simulink library "inp"  (R2024a)
settings: Solver=VariableStepAuto  StartTime=0.0  StopTime=10.0  RelTol=1e-3
undefined symbols (not defined in the file): C_TASK_5MS_S, TRUE
libraries: FVT_lib x54, hcu_lib x1
(part 2 of 2)

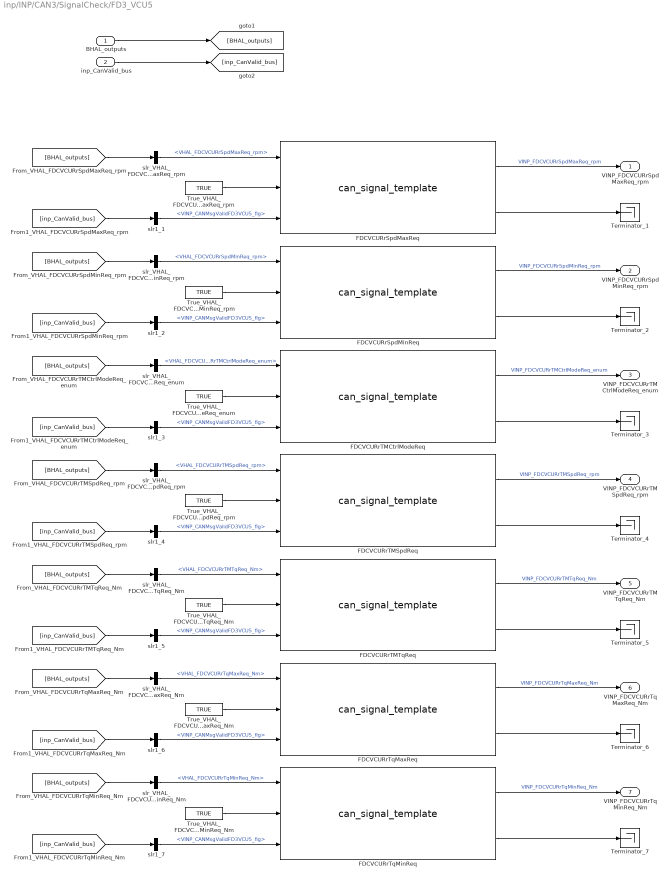
== system inp/INP/CAN3/SignalCheck/FD3_VCU5 ==
  BHAL_outputs : Inport
  inp_CanValid_bus : Inport  Port=2
  FDCVCURrSpdMaxReq : FVT_lib/inp/can_signal_template  SystemSampleTime=-1  VariantActivationTime=update diagram  AllowFlexibleInterface=on  Latency=0  AutoFrameSizeCalculation=off
      link override defval: Value=KINP_FDCVCURrSpdMaxReq_rpm_defval
      link override ovrdflg: Value=KINP_FDCVCURrSpdMaxReq_rpm_ovrdflg
      link override ovrdval: Value=KINP_FDCVCURrSpdMaxReq_rpm_ovrdval
  FDCVCURrSpdMinReq : FVT_lib/inp/can_signal_template  SystemSampleTime=-1  VariantActivationTime=update diagram  AllowFlexibleInterface=on  Latency=0  AutoFrameSizeCalculation=off
      link override defval: Value=KINP_FDCVCURrSpdMinReq_rpm_defval
      link override ovrdflg: Value=KINP_FDCVCURrSpdMinReq_rpm_ovrdflg
      link override ovrdval: Value=KINP_FDCVCURrSpdMinReq_rpm_ovrdval
  FDCVCURrTMCtrlModeReq : FVT_lib/inp/can_signal_template  SystemSampleTime=-1  VariantActivationTime=update diagram  AllowFlexibleInterface=on  Latency=0  AutoFrameSizeCalculation=off
      link override defval: Value=KINP_FDCVCURrTMCtrlModeReq_enum_defval
      link override ovrdflg: Value=KINP_FDCVCURrTMCtrlModeReq_enum_ovrdflg
      link override ovrdval: Value=KINP_FDCVCURrTMCtrlModeReq_enum_ovrdval
  FDCVCURrTMSpdReq : FVT_lib/inp/can_signal_template  SystemSampleTime=-1  VariantActivationTime=update diagram  AllowFlexibleInterface=on  Latency=0  AutoFrameSizeCalculation=off
      link override defval: Value=KINP_FDCVCURrTMSpdReq_rpm_defval
      link override ovrdflg: Value=KINP_FDCVCURrTMSpdReq_rpm_ovrdflg
      link override ovrdval: Value=KINP_FDCVCURrTMSpdReq_rpm_ovrdval
  FDCVCURrTMTqReq : FVT_lib/inp/can_signal_template  SystemSampleTime=-1  VariantActivationTime=update diagram  AllowFlexibleInterface=on  Latency=0  AutoFrameSizeCalculation=off
      link override defval: Value=KINP_FDCVCURrTMTqReq_Nm_defval
      link override ovrdflg: Value=KINP_FDCVCURrTMTqReq_Nm_ovrdflg
      link override ovrdval: Value=KINP_FDCVCURrTMTqReq_Nm_ovrdval
  FDCVCURrTqMaxReq : FVT_lib/inp/can_signal_template  SystemSampleTime=-1  VariantActivationTime=update diagram  AllowFlexibleInterface=on  Latency=0  AutoFrameSizeCalculation=off
      link override defval: Value=KINP_FDCVCURrTqMaxReq_Nm_defval
      link override ovrdflg: Value=KINP_FDCVCURrTqMaxReq_Nm_ovrdflg
      link override ovrdval: Value=KINP_FDCVCURrTqMaxReq_Nm_ovrdval
  FDCVCURrTqMinReq : FVT_lib/inp/can_signal_template  SystemSampleTime=-1  VariantActivationTime=update diagram  AllowFlexibleInterface=on  Latency=0  AutoFrameSizeCalculation=off
      link override defval: Value=KINP_FDCVCURrTqMinReq_Nm_defval
      link override ovrdflg: Value=KINP_FDCVCURrTqMinReq_Nm_ovrdflg
      link override ovrdval: Value=KINP_FDCVCURrTqMinReq_Nm_ovrdval
  Terminator_{1..7} (7 alike) : Terminator
  True_VHAL_FDCVCURrSpdMaxReq_rpm : Constant  Value=TRUE  OutDataTypeStr=boolean
  True_VHAL_FDCVCURrSpdMinReq_rpm : Constant  Value=TRUE  OutDataTypeStr=boolean
  True_VHAL_FDCVCURrTMCtrlModeReq_enum : Constant  Value=TRUE  OutDataTypeStr=boolean
  True_VHAL_FDCVCURrTMSpdReq_rpm : Constant  Value=TRUE  OutDataTypeStr=boolean
  True_VHAL_FDCVCURrTMTqReq_Nm : Constant  Value=TRUE  OutDataTypeStr=boolean
  True_VHAL_FDCVCURrTqMaxReq_Nm : Constant  Value=TRUE  OutDataTypeStr=boolean
  True_VHAL_FDCVCURrTqMinReq_Nm : Constant  Value=TRUE  OutDataTypeStr=boolean
  slr1_{1..7} (7 alike) : BusSelector  OutputSignals=VINP_CANMsgValidFD3VCU5_flg
  slr_VHAL_FDCVCURrSpdMaxReq_rpm : BusSelector  OutputSignals=VHAL_FDCVCURrSpdMaxReq_rpm
  slr_VHAL_FDCVCURrSpdMinReq_rpm : BusSelector  OutputSignals=VHAL_FDCVCURrSpdMinReq_rpm
  slr_VHAL_FDCVCURrTMCtrlModeReq_enum : BusSelector  OutputSignals=VHAL_FDCVCURrTMCtrlModeReq_enum
  slr_VHAL_FDCVCURrTMSpdReq_rpm : BusSelector  OutputSignals=VHAL_FDCVCURrTMSpdReq_rpm
  slr_VHAL_FDCVCURrTMTqReq_Nm : BusSelector  OutputSignals=VHAL_FDCVCURrTMTqReq_Nm
  slr_VHAL_FDCVCURrTqMaxReq_Nm : BusSelector  OutputSignals=VHAL_FDCVCURrTqMaxReq_Nm
  slr_VHAL_FDCVCURrTqMinReq_Nm : BusSelector  OutputSignals=VHAL_FDCVCURrTqMinReq_Nm
  VINP_FDCVCURrSpdMaxReq_rpm : Outport
  VINP_FDCVCURrSpdMinReq_rpm : Outport  Port=2
  VINP_FDCVCURrTMCtrlModeReq_enum : Outport  Port=3
  VINP_FDCVCURrTMSpdReq_rpm : Outport  Port=4
  VINP_FDCVCURrTMTqReq_Nm : Outport  Port=5
  VINP_FDCVCURrTqMaxReq_Nm : Outport  Port=6
  VINP_FDCVCURrTqMinReq_Nm : Outport  Port=7
  wires:
  BHAL_outputs/1 -> [BHAL_outputs]
  inp_CanValid_bus/1 -> [inp_CanValid_bus]
  [BHAL_outputs] -> slr_VHAL_FDCVCURrSpdMaxReq_rpm/1
  slr_VHAL_FDCVCURrSpdMaxReq_rpm/1 -> FDCVCURrSpdMaxReq/1  "<VHAL_FDCVCURrSpdMaxReq_rpm>"
  True_VHAL_FDCVCURrSpdMaxReq_rpm/1 -> FDCVCURrSpdMaxReq/2
  [inp_CanValid_bus] -> slr1_1/1
  slr1_1/1 -> FDCVCURrSpdMaxReq/3  "<VINP_CANMsgValidFD3VCU5_flg>"
  FDCVCURrSpdMaxReq/1 -> VINP_FDCVCURrSpdMaxReq_rpm/1  "VINP_FDCVCURrSpdMaxReq_rpm"
  FDCVCURrSpdMaxReq/2 -> Terminator_1/1
  [BHAL_outputs] -> slr_VHAL_FDCVCURrSpdMinReq_rpm/1
  slr_VHAL_FDCVCURrSpdMinReq_rpm/1 -> FDCVCURrSpdMinReq/1  "<VHAL_FDCVCURrSpdMinReq_rpm>"
  True_VHAL_FDCVCURrSpdMinReq_rpm/1 -> FDCVCURrSpdMinReq/2
  [inp_CanValid_bus] -> slr1_2/1
  slr1_2/1 -> FDCVCURrSpdMinReq/3  "<VINP_CANMsgValidFD3VCU5_flg>"
  FDCVCURrSpdMinReq/1 -> VINP_FDCVCURrSpdMinReq_rpm/1  "VINP_FDCVCURrSpdMinReq_rpm"
  FDCVCURrSpdMinReq/2 -> Terminator_2/1
  [BHAL_outputs] -> slr_VHAL_FDCVCURrTMCtrlModeReq_enum/1
  slr_VHAL_FDCVCURrTMCtrlModeReq_enum/1 -> FDCVCURrTMCtrlModeReq/1  "<VHAL_FDCVCURrTMCtrlModeReq_enum>"
  True_VHAL_FDCVCURrTMCtrlModeReq_enum/1 -> FDCVCURrTMCtrlModeReq/2
  [inp_CanValid_bus] -> slr1_3/1
  slr1_3/1 -> FDCVCURrTMCtrlModeReq/3  "<VINP_CANMsgValidFD3VCU5_flg>"
  FDCVCURrTMCtrlModeReq/1 -> VINP_FDCVCURrTMCtrlModeReq_enum/1  "VINP_FDCVCURrTMCtrlModeReq_enum"
  FDCVCURrTMCtrlModeReq/2 -> Terminator_3/1
  [BHAL_outputs] -> slr_VHAL_FDCVCURrTMSpdReq_rpm/1
  slr_VHAL_FDCVCURrTMSpdReq_rpm/1 -> FDCVCURrTMSpdReq/1  "<VHAL_FDCVCURrTMSpdReq_rpm>"
  True_VHAL_FDCVCURrTMSpdReq_rpm/1 -> FDCVCURrTMSpdReq/2
  [inp_CanValid_bus] -> slr1_4/1
  slr1_4/1 -> FDCVCURrTMSpdReq/3  "<VINP_CANMsgValidFD3VCU5_flg>"
  FDCVCURrTMSpdReq/1 -> VINP_FDCVCURrTMSpdReq_rpm/1  "VINP_FDCVCURrTMSpdReq_rpm"
  FDCVCURrTMSpdReq/2 -> Terminator_4/1
  [BHAL_outputs] -> slr_VHAL_FDCVCURrTMTqReq_Nm/1
  slr_VHAL_FDCVCURrTMTqReq_Nm/1 -> FDCVCURrTMTqReq/1  "<VHAL_FDCVCURrTMTqReq_Nm>"
  True_VHAL_FDCVCURrTMTqReq_Nm/1 -> FDCVCURrTMTqReq/2
  [inp_CanValid_bus] -> slr1_5/1
  slr1_5/1 -> FDCVCURrTMTqReq/3  "<VINP_CANMsgValidFD3VCU5_flg>"
  FDCVCURrTMTqReq/1 -> VINP_FDCVCURrTMTqReq_Nm/1  "VINP_FDCVCURrTMTqReq_Nm"
  FDCVCURrTMTqReq/2 -> Terminator_5/1
  [BHAL_outputs] -> slr_VHAL_FDCVCURrTqMaxReq_Nm/1
  slr_VHAL_FDCVCURrTqMaxReq_Nm/1 -> FDCVCURrTqMaxReq/1  "<VHAL_FDCVCURrTqMaxReq_Nm>"
  True_VHAL_FDCVCURrTqMaxReq_Nm/1 -> FDCVCURrTqMaxReq/2
  [inp_CanValid_bus] -> slr1_6/1
  slr1_6/1 -> FDCVCURrTqMaxReq/3  "<VINP_CANMsgValidFD3VCU5_flg>"
  FDCVCURrTqMaxReq/1 -> VINP_FDCVCURrTqMaxReq_Nm/1  "VINP_FDCVCURrTqMaxReq_Nm"
  FDCVCURrTqMaxReq/2 -> Terminator_6/1
  [BHAL_outputs] -> slr_VHAL_FDCVCURrTqMinReq_Nm/1
  slr_VHAL_FDCVCURrTqMinReq_Nm/1 -> FDCVCURrTqMinReq/1  "<VHAL_FDCVCURrTqMinReq_Nm>"
  True_VHAL_FDCVCURrTqMinReq_Nm/1 -> FDCVCURrTqMinReq/2
  [inp_CanValid_bus] -> slr1_7/1
  slr1_7/1 -> FDCVCURrTqMinReq/3  "<VINP_CANMsgValidFD3VCU5_flg>"
  FDCVCURrTqMinReq/1 -> VINP_FDCVCURrTqMinReq_Nm/1  "VINP_FDCVCURrTqMinReq_Nm"
  FDCVCURrTqMinReq/2 -> Terminator_7/1

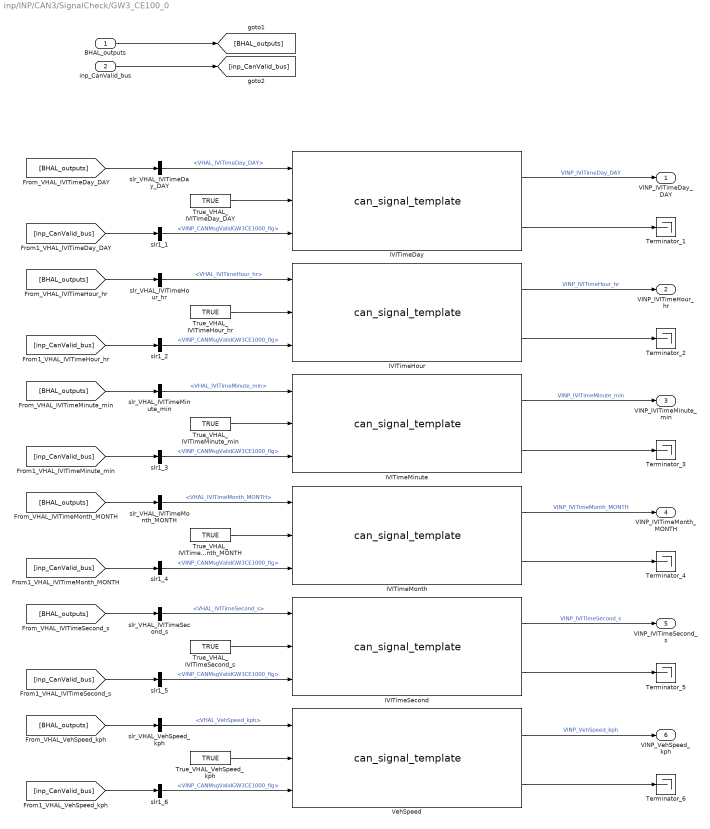
== system inp/INP/CAN3/SignalCheck/GW3_CE100_0 ==
  BHAL_outputs : Inport
  inp_CanValid_bus : Inport  Port=2
  IVITimeDay : FVT_lib/inp/can_signal_template  SystemSampleTime=-1  VariantActivationTime=update diagram  AllowFlexibleInterface=on  Latency=0  AutoFrameSizeCalculation=off
      link override defval: Value=KINP_IVITimeDay_DAY_defval
      link override ovrdflg: Value=KINP_IVITimeDay_DAY_ovrdflg
      link override ovrdval: Value=KINP_IVITimeDay_DAY_ovrdval
  IVITimeHour : FVT_lib/inp/can_signal_template  SystemSampleTime=-1  VariantActivationTime=update diagram  AllowFlexibleInterface=on  Latency=0  AutoFrameSizeCalculation=off
      link override defval: Value=KINP_IVITimeHour_hr_defval
      link override ovrdflg: Value=KINP_IVITimeHour_hr_ovrdflg
      link override ovrdval: Value=KINP_IVITimeHour_hr_ovrdval
  IVITimeMinute : FVT_lib/inp/can_signal_template  SystemSampleTime=-1  VariantActivationTime=update diagram  AllowFlexibleInterface=on  Latency=0  AutoFrameSizeCalculation=off
      link override defval: Value=KINP_IVITimeMinute_min_defval
      link override ovrdflg: Value=KINP_IVITimeMinute_min_ovrdflg
      link override ovrdval: Value=KINP_IVITimeMinute_min_ovrdval
  IVITimeMonth : FVT_lib/inp/can_signal_template  SystemSampleTime=-1  VariantActivationTime=update diagram  AllowFlexibleInterface=on  Latency=0  AutoFrameSizeCalculation=off
      link override defval: Value=KINP_IVITimeMonth_MONTH_defval
      link override ovrdflg: Value=KINP_IVITimeMonth_MONTH_ovrdflg
      link override ovrdval: Value=KINP_IVITimeMonth_MONTH_ovrdval
  IVITimeSecond : FVT_lib/inp/can_signal_template  SystemSampleTime=-1  VariantActivationTime=update diagram  AllowFlexibleInterface=on  Latency=0  AutoFrameSizeCalculation=off
      link override defval: Value=KINP_IVITimeSecond_s_defval
      link override ovrdflg: Value=KINP_IVITimeSecond_s_ovrdflg
      link override ovrdval: Value=KINP_IVITimeSecond_s_ovrdval
  Terminator_{1..6} (6 alike) : Terminator
  True_VHAL_IVITimeDay_DAY : Constant  Value=TRUE  OutDataTypeStr=boolean
  True_VHAL_IVITimeHour_hr : Constant  Value=TRUE  OutDataTypeStr=boolean
  True_VHAL_IVITimeMinute_min : Constant  Value=TRUE  OutDataTypeStr=boolean
  True_VHAL_IVITimeMonth_MONTH : Constant  Value=TRUE  OutDataTypeStr=boolean
  True_VHAL_IVITimeSecond_s : Constant  Value=TRUE  OutDataTypeStr=boolean
  True_VHAL_VehSpeed_kph : Constant  Value=TRUE  OutDataTypeStr=boolean
  VehSpeed : FVT_lib/inp/can_signal_template  SystemSampleTime=-1  VariantActivationTime=update diagram  AllowFlexibleInterface=on  Latency=0  AutoFrameSizeCalculation=off
      link override defval: Value=KINP_VehSpeed_kph_defval
      link override ovrdflg: Value=KINP_VehSpeed_kph_ovrdflg
      link override ovrdval: Value=KINP_VehSpeed_kph_ovrdval
  slr1_{1..6} (6 alike) : BusSelector  OutputSignals=VINP_CANMsgValidGW3CE1000_flg
  slr_VHAL_IVITimeDay_DAY : BusSelector  OutputSignals=VHAL_IVITimeDay_DAY
  slr_VHAL_IVITimeHour_hr : BusSelector  OutputSignals=VHAL_IVITimeHour_hr
  slr_VHAL_IVITimeMinute_min : BusSelector  OutputSignals=VHAL_IVITimeMinute_min
  slr_VHAL_IVITimeMonth_MONTH : BusSelector  OutputSignals=VHAL_IVITimeMonth_MONTH
  slr_VHAL_IVITimeSecond_s : BusSelector  OutputSignals=VHAL_IVITimeSecond_s
  slr_VHAL_VehSpeed_kph : BusSelector  OutputSignals=VHAL_VehSpeed_kph
  VINP_IVITimeDay_DAY : Outport
  VINP_IVITimeHour_hr : Outport  Port=2
  VINP_IVITimeMinute_min : Outport  Port=3
  VINP_IVITimeMonth_MONTH : Outport  Port=4
  VINP_IVITimeSecond_s : Outport  Port=5
  VINP_VehSpeed_kph : Outport  Port=6
  wires:
  BHAL_outputs/1 -> [BHAL_outputs]
  inp_CanValid_bus/1 -> [inp_CanValid_bus]
  [BHAL_outputs] -> slr_VHAL_IVITimeDay_DAY/1
  slr_VHAL_IVITimeDay_DAY/1 -> IVITimeDay/1  "<VHAL_IVITimeDay_DAY>"
  True_VHAL_IVITimeDay_DAY/1 -> IVITimeDay/2
  [inp_CanValid_bus] -> slr1_1/1
  slr1_1/1 -> IVITimeDay/3  "<VINP_CANMsgValidGW3CE1000_flg>"
  IVITimeDay/1 -> VINP_IVITimeDay_DAY/1  "VINP_IVITimeDay_DAY"
  IVITimeDay/2 -> Terminator_1/1
  [BHAL_outputs] -> slr_VHAL_IVITimeHour_hr/1
  slr_VHAL_IVITimeHour_hr/1 -> IVITimeHour/1  "<VHAL_IVITimeHour_hr>"
  True_VHAL_IVITimeHour_hr/1 -> IVITimeHour/2
  [inp_CanValid_bus] -> slr1_2/1
  slr1_2/1 -> IVITimeHour/3  "<VINP_CANMsgValidGW3CE1000_flg>"
  IVITimeHour/1 -> VINP_IVITimeHour_hr/1  "VINP_IVITimeHour_hr"
  IVITimeHour/2 -> Terminator_2/1
  [BHAL_outputs] -> slr_VHAL_IVITimeMinute_min/1
  slr_VHAL_IVITimeMinute_min/1 -> IVITimeMinute/1  "<VHAL_IVITimeMinute_min>"
  True_VHAL_IVITimeMinute_min/1 -> IVITimeMinute/2
  [inp_CanValid_bus] -> slr1_3/1
  slr1_3/1 -> IVITimeMinute/3  "<VINP_CANMsgValidGW3CE1000_flg>"
  IVITimeMinute/1 -> VINP_IVITimeMinute_min/1  "VINP_IVITimeMinute_min"
  IVITimeMinute/2 -> Terminator_3/1
  [BHAL_outputs] -> slr_VHAL_IVITimeMonth_MONTH/1
  slr_VHAL_IVITimeMonth_MONTH/1 -> IVITimeMonth/1  "<VHAL_IVITimeMonth_MONTH>"
  True_VHAL_IVITimeMonth_MONTH/1 -> IVITimeMonth/2
  [inp_CanValid_bus] -> slr1_4/1
  slr1_4/1 -> IVITimeMonth/3  "<VINP_CANMsgValidGW3CE1000_flg>"
  IVITimeMonth/1 -> VINP_IVITimeMonth_MONTH/1  "VINP_IVITimeMonth_MONTH"
  IVITimeMonth/2 -> Terminator_4/1
  [BHAL_outputs] -> slr_VHAL_IVITimeSecond_s/1
  slr_VHAL_IVITimeSecond_s/1 -> IVITimeSecond/1  "<VHAL_IVITimeSecond_s>"
  True_VHAL_IVITimeSecond_s/1 -> IVITimeSecond/2
  [inp_CanValid_bus] -> slr1_5/1
  slr1_5/1 -> IVITimeSecond/3  "<VINP_CANMsgValidGW3CE1000_flg>"
  IVITimeSecond/1 -> VINP_IVITimeSecond_s/1  "VINP_IVITimeSecond_s"
  IVITimeSecond/2 -> Terminator_5/1
  [BHAL_outputs] -> slr_VHAL_VehSpeed_kph/1
  slr_VHAL_VehSpeed_kph/1 -> VehSpeed/1  "<VHAL_VehSpeed_kph>"
  True_VHAL_VehSpeed_kph/1 -> VehSpeed/2
  [inp_CanValid_bus] -> slr1_6/1
  slr1_6/1 -> VehSpeed/3  "<VINP_CANMsgValidGW3CE1000_flg>"
  VehSpeed/1 -> VINP_VehSpeed_kph/1  "VINP_VehSpeed_kph"
  VehSpeed/2 -> Terminator_6/1

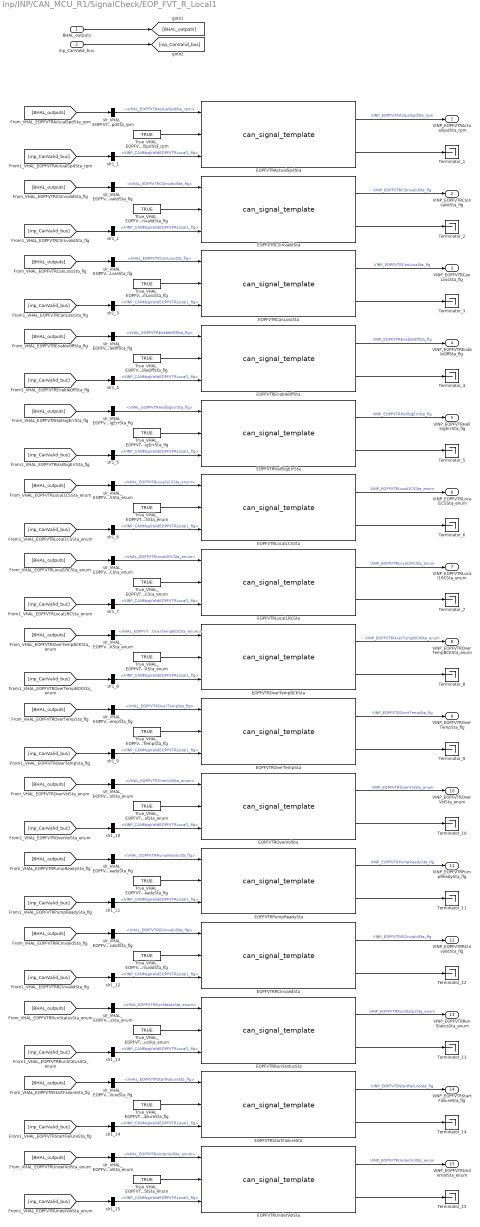
== system inp/INP/CAN_MCU_R1/SignalCheck/EOP_FVT_R_Local1 ==
  BHAL_outputs : Inport
  inp_CanValid_bus : Inport  Port=2
  EOPFVTRActualSpdSta : FVT_lib/inp/can_signal_template  SystemSampleTime=-1  VariantActivationTime=update diagram  AllowFlexibleInterface=on  Latency=0  AutoFrameSizeCalculation=off
      link override defval: Value=KINP_EOPFVTRActualSpdSta_rpm_defval
      link override ovrdflg: Value=KINP_EOPFVTRActualSpdSta_rpm_ovrdflg
      link override ovrdval: Value=KINP_EOPFVTRActualSpdSta_rpm_ovrdval
  EOPFVTRCSInvalidSta : FVT_lib/inp/can_signal_template  SystemSampleTime=-1  VariantActivationTime=update diagram  AllowFlexibleInterface=on  Latency=0  AutoFrameSizeCalculation=off
      link override defval: Value=KINP_EOPFVTRCSInvalidSta_flg_defval
      link override ovrdflg: Value=KINP_EOPFVTRCSInvalidSta_flg_ovrdflg
      link override ovrdval: Value=KINP_EOPFVTRCSInvalidSta_flg_ovrdval
  EOPFVTRCanLossSta : FVT_lib/inp/can_signal_template  SystemSampleTime=-1  VariantActivationTime=update diagram  AllowFlexibleInterface=on  Latency=0  AutoFrameSizeCalculation=off
      link override defval: Value=KINP_EOPFVTRCanLossSta_flg_defval
      link override ovrdflg: Value=KINP_EOPFVTRCanLossSta_flg_ovrdflg
      link override ovrdval: Value=KINP_EOPFVTRCanLossSta_flg_ovrdval
  EOPFVTREnableOffSta : FVT_lib/inp/can_signal_template  SystemSampleTime=-1  VariantActivationTime=update diagram  AllowFlexibleInterface=on  Latency=0  AutoFrameSizeCalculation=off
      link override defval: Value=KINP_EOPFVTREnableOffSta_flg_defval
      link override ovrdflg: Value=KINP_EOPFVTREnableOffSta_flg_ovrdflg
      link override ovrdval: Value=KINP_EOPFVTREnableOffSta_flg_ovrdval
  EOPFVTRHallSigErrSta : FVT_lib/inp/can_signal_template  SystemSampleTime=-1  VariantActivationTime=update diagram  AllowFlexibleInterface=on  Latency=0  AutoFrameSizeCalculation=off
      link override defval: Value=KINP_EOPFVTRHallSigErrSta_flg_defval
      link override ovrdflg: Value=KINP_EOPFVTRHallSigErrSta_flg_ovrdflg
      link override ovrdval: Value=KINP_EOPFVTRHallSigErrSta_flg_ovrdval
  EOPFVTRLocal1CSSta : FVT_lib/inp/can_signal_template  SystemSampleTime=-1  VariantActivationTime=update diagram  AllowFlexibleInterface=on  Latency=0  AutoFrameSizeCalculation=off
      link override defval: Value=KINP_EOPFVTRLocal1CSSta_enum_defval
      link override ovrdflg: Value=KINP_EOPFVTRLocal1CSSta_enum_ovrdflg
      link override ovrdval: Value=KINP_EOPFVTRLocal1CSSta_enum_ovrdval
  EOPFVTRLocal1RCSta : FVT_lib/inp/can_signal_template  SystemSampleTime=-1  VariantActivationTime=update diagram  AllowFlexibleInterface=on  Latency=0  AutoFrameSizeCalculation=off
      link override defval: Value=KINP_EOPFVTRLocal1RCSta_enum_defval
      link override ovrdflg: Value=KINP_EOPFVTRLocal1RCSta_enum_ovrdflg
      link override ovrdval: Value=KINP_EOPFVTRLocal1RCSta_enum_ovrdval
  EOPFVTROverTempBCKSta : FVT_lib/inp/can_signal_template  SystemSampleTime=-1  VariantActivationTime=update diagram  AllowFlexibleInterface=on  Latency=0  AutoFrameSizeCalculation=off
      link override defval: Value=KINP_EOPFVTROverTempBCKSta_enum_defval
      link override ovrdflg: Value=KINP_EOPFVTROverTempBCKSta_enum_ovrdflg
      link override ovrdval: Value=KINP_EOPFVTROverTempBCKSta_enum_ovrdval
  EOPFVTROverTempSta : FVT_lib/inp/can_signal_template  SystemSampleTime=-1  VariantActivationTime=update diagram  AllowFlexibleInterface=on  Latency=0  AutoFrameSizeCalculation=off
      link override defval: Value=KINP_EOPFVTROverTempSta_flg_defval
      link override ovrdflg: Value=KINP_EOPFVTROverTempSta_flg_ovrdflg
      link override ovrdval: Value=KINP_EOPFVTROverTempSta_flg_ovrdval
  EOPFVTROverVolSta : FVT_lib/inp/can_signal_template  SystemSampleTime=-1  VariantActivationTime=update diagram  AllowFlexibleInterface=on  Latency=0  AutoFrameSizeCalculation=off
      link override defval: Value=KINP_EOPFVTROverVolSta_enum_defval
      link override ovrdflg: Value=KINP_EOPFVTROverVolSta_enum_ovrdflg
      link override ovrdval: Value=KINP_EOPFVTROverVolSta_enum_ovrdval
  EOPFVTRPumpReadySta : FVT_lib/inp/can_signal_template  SystemSampleTime=-1  VariantActivationTime=update diagram  AllowFlexibleInterface=on  Latency=0  AutoFrameSizeCalculation=off
      link override defval: Value=KINP_EOPFVTRPumpReadySta_flg_defval
      link override ovrdflg: Value=KINP_EOPFVTRPumpReadySta_flg_ovrdflg
      link override ovrdval: Value=KINP_EOPFVTRPumpReadySta_flg_ovrdval
  EOPFVTRRCInvalidSta : FVT_lib/inp/can_signal_template  SystemSampleTime=-1  VariantActivationTime=update diagram  AllowFlexibleInterface=on  Latency=0  AutoFrameSizeCalculation=off
      link override defval: Value=KINP_EOPFVTRRCInvalidSta_flg_defval
      link override ovrdflg: Value=KINP_EOPFVTRRCInvalidSta_flg_ovrdflg
      link override ovrdval: Value=KINP_EOPFVTRRCInvalidSta_flg_ovrdval
  EOPFVTRRunStatusSta : FVT_lib/inp/can_signal_template  SystemSampleTime=-1  VariantActivationTime=update diagram  AllowFlexibleInterface=on  Latency=0  AutoFrameSizeCalculation=off
      link override defval: Value=KINP_EOPFVTRRunStatusSta_enum_defval
      link override ovrdflg: Value=KINP_EOPFVTRRunStatusSta_enum_ovrdflg
      link override ovrdval: Value=KINP_EOPFVTRRunStatusSta_enum_ovrdval
  EOPFVTRStartFailureSta : FVT_lib/inp/can_signal_template  SystemSampleTime=-1  VariantActivationTime=update diagram  AllowFlexibleInterface=on  Latency=0  AutoFrameSizeCalculation=off
      link override defval: Value=KINP_EOPFVTRStartFailureSta_flg_defval
      link override ovrdflg: Value=KINP_EOPFVTRStartFailureSta_flg_ovrdflg
      link override ovrdval: Value=KINP_EOPFVTRStartFailureSta_flg_ovrdval
  EOPFVTRUnderVolSta : FVT_lib/inp/can_signal_template  SystemSampleTime=-1  VariantActivationTime=update diagram  AllowFlexibleInterface=on  Latency=0  AutoFrameSizeCalculation=off
      link override defval: Value=KINP_EOPFVTRUnderVolSta_enum_defval
      link override ovrdflg: Value=KINP_EOPFVTRUnderVolSta_enum_ovrdflg
      link override ovrdval: Value=KINP_EOPFVTRUnderVolSta_enum_ovrdval
  Terminator_{1..15} (15 alike) : Terminator
  True_VHAL_EOPFVTRActualSpdSta_rpm : Constant  Value=TRUE  OutDataTypeStr=boolean
  True_VHAL_EOPFVTRCSInvalidSta_flg : Constant  Value=TRUE  OutDataTypeStr=boolean
  True_VHAL_EOPFVTRCanLossSta_flg : Constant  Value=TRUE  OutDataTypeStr=boolean
  True_VHAL_EOPFVTREnableOffSta_flg : Constant  Value=TRUE  OutDataTypeStr=boolean
  True_VHAL_EOPFVTRHallSigErrSta_flg : Constant  Value=TRUE  OutDataTypeStr=boolean
  True_VHAL_EOPFVTRLocal1CSSta_enum : Constant  Value=TRUE  OutDataTypeStr=boolean
  True_VHAL_EOPFVTRLocal1RCSta_enum : Constant  Value=TRUE  OutDataTypeStr=boolean
  True_VHAL_EOPFVTROverTempBCKSta_enum : Constant  Value=TRUE  OutDataTypeStr=boolean
  True_VHAL_EOPFVTROverTempSta_flg : Constant  Value=TRUE  OutDataTypeStr=boolean
  True_VHAL_EOPFVTROverVolSta_enum : Constant  Value=TRUE  OutDataTypeStr=boolean
  True_VHAL_EOPFVTRPumpReadySta_flg : Constant  Value=TRUE  OutDataTypeStr=boolean
  True_VHAL_EOPFVTRRCInvalidSta_flg : Constant  Value=TRUE  OutDataTypeStr=boolean
  True_VHAL_EOPFVTRRunStatusSta_enum : Constant  Value=TRUE  OutDataTypeStr=boolean
  True_VHAL_EOPFVTRStartFailureSta_flg : Constant  Value=TRUE  OutDataTypeStr=boolean
  True_VHAL_EOPFVTRUnderVolSta_enum : Constant  Value=TRUE  OutDataTypeStr=boolean
  slr1_{1..15} (15 alike) : BusSelector  OutputSignals=VINP_CANMsgValidEOPFVTRLocal1_flg
  slr_VHAL_EOPFVTRActualSpdSta_rpm : BusSelector  OutputSignals=VHAL_EOPFVTRActualSpdSta_rpm
  slr_VHAL_EOPFVTRCSInvalidSta_flg : BusSelector  OutputSignals=VHAL_EOPFVTRCSInvalidSta_flg
  slr_VHAL_EOPFVTRCanLossSta_flg : BusSelector  OutputSignals=VHAL_EOPFVTRCanLossSta_flg
  slr_VHAL_EOPFVTREnableOffSta_flg : BusSelector  OutputSignals=VHAL_EOPFVTREnableOffSta_flg
  slr_VHAL_EOPFVTRHallSigErrSta_flg : BusSelector  OutputSignals=VHAL_EOPFVTRHallSigErrSta_flg
  slr_VHAL_EOPFVTRLocal1CSSta_enum : BusSelector  OutputSignals=VHAL_EOPFVTRLocal1CSSta_enum
  slr_VHAL_EOPFVTRLocal1RCSta_enum : BusSelector  OutputSignals=VHAL_EOPFVTRLocal1RCSta_enum
  slr_VHAL_EOPFVTROverTempBCKSta_enum : BusSelector  OutputSignals=VHAL_EOPFVTROverTempBCKSta_enum
  slr_VHAL_EOPFVTROverTempSta_flg : BusSelector  OutputSignals=VHAL_EOPFVTROverTempSta_flg
  slr_VHAL_EOPFVTROverVolSta_enum : BusSelector  OutputSignals=VHAL_EOPFVTROverVolSta_enum
  slr_VHAL_EOPFVTRPumpReadySta_flg : BusSelector  OutputSignals=VHAL_EOPFVTRPumpReadySta_flg
  slr_VHAL_EOPFVTRRCInvalidSta_flg : BusSelector  OutputSignals=VHAL_EOPFVTRRCInvalidSta_flg
  slr_VHAL_EOPFVTRRunStatusSta_enum : BusSelector  OutputSignals=VHAL_EOPFVTRRunStatusSta_enum
  slr_VHAL_EOPFVTRStartFailureSta_flg : BusSelector  OutputSignals=VHAL_EOPFVTRStartFailureSta_flg
  slr_VHAL_EOPFVTRUnderVolSta_enum : BusSelector  OutputSignals=VHAL_EOPFVTRUnderVolSta_enum
  VINP_EOPFVTRActualSpdSta_rpm : Outport
  VINP_EOPFVTRCSInvalidSta_flg : Outport  Port=2
  VINP_EOPFVTRCanLossSta_flg : Outport  Port=3
  VINP_EOPFVTREnableOffSta_flg : Outport  Port=4
  VINP_EOPFVTRHallSigErrSta_flg : Outport  Port=5
  VINP_EOPFVTRLocal1CSSta_enum : Outport  Port=6
  VINP_EOPFVTRLocal1RCSta_enum : Outport  Port=7
  VINP_EOPFVTROverTempBCKSta_enum : Outport  Port=8
  VINP_EOPFVTROverTempSta_flg : Outport  Port=9
  VINP_EOPFVTROverVolSta_enum : Outport  Port=10
  VINP_EOPFVTRPumpReadySta_flg : Outport  Port=11
  VINP_EOPFVTRRCInvalidSta_flg : Outport  Port=12
  VINP_EOPFVTRRunStatusSta_enum : Outport  Port=13
  VINP_EOPFVTRStartFailureSta_flg : Outport  Port=14
  VINP_EOPFVTRUnderVolSta_enum : Outport  Port=15
  wires:
  BHAL_outputs/1 -> [BHAL_outputs]
  inp_CanValid_bus/1 -> [inp_CanValid_bus]
  [BHAL_outputs] -> slr_VHAL_EOPFVTRActualSpdSta_rpm/1
  slr_VHAL_EOPFVTRActualSpdSta_rpm/1 -> EOPFVTRActualSpdSta/1  "<VHAL_EOPFVTRActualSpdSta_rpm>"
  True_VHAL_EOPFVTRActualSpdSta_rpm/1 -> EOPFVTRActualSpdSta/2
  [inp_CanValid_bus] -> slr1_1/1
  slr1_1/1 -> EOPFVTRActualSpdSta/3  "<VINP_CANMsgValidEOPFVTRLocal1_flg>"
  EOPFVTRActualSpdSta/1 -> VINP_EOPFVTRActualSpdSta_rpm/1  "VINP_EOPFVTRActualSpdSta_rpm"
  EOPFVTRActualSpdSta/2 -> Terminator_1/1
  [BHAL_outputs] -> slr_VHAL_EOPFVTRCSInvalidSta_flg/1
  slr_VHAL_EOPFVTRCSInvalidSta_flg/1 -> EOPFVTRCSInvalidSta/1  "<VHAL_EOPFVTRCSInvalidSta_flg>"
  True_VHAL_EOPFVTRCSInvalidSta_flg/1 -> EOPFVTRCSInvalidSta/2
  [inp_CanValid_bus] -> slr1_2/1
  slr1_2/1 -> EOPFVTRCSInvalidSta/3  "<VINP_CANMsgValidEOPFVTRLocal1_flg>"
  EOPFVTRCSInvalidSta/1 -> VINP_EOPFVTRCSInvalidSta_flg/1  "VINP_EOPFVTRCSInvalidSta_flg"
  EOPFVTRCSInvalidSta/2 -> Terminator_2/1
  [BHAL_outputs] -> slr_VHAL_EOPFVTRCanLossSta_flg/1
  slr_VHAL_EOPFVTRCanLossSta_flg/1 -> EOPFVTRCanLossSta/1  "<VHAL_EOPFVTRCanLossSta_flg>"
  True_VHAL_EOPFVTRCanLossSta_flg/1 -> EOPFVTRCanLossSta/2
  [inp_CanValid_bus] -> slr1_3/1
  slr1_3/1 -> EOPFVTRCanLossSta/3  "<VINP_CANMsgValidEOPFVTRLocal1_flg>"
  EOPFVTRCanLossSta/1 -> VINP_EOPFVTRCanLossSta_flg/1  "VINP_EOPFVTRCanLossSta_flg"
  EOPFVTRCanLossSta/2 -> Terminator_3/1
  [BHAL_outputs] -> slr_VHAL_EOPFVTREnableOffSta_flg/1
  slr_VHAL_EOPFVTREnableOffSta_flg/1 -> EOPFVTREnableOffSta/1  "<VHAL_EOPFVTREnableOffSta_flg>"
  True_VHAL_EOPFVTREnableOffSta_flg/1 -> EOPFVTREnableOffSta/2
  [inp_CanValid_bus] -> slr1_4/1
  slr1_4/1 -> EOPFVTREnableOffSta/3  "<VINP_CANMsgValidEOPFVTRLocal1_flg>"
  EOPFVTREnableOffSta/1 -> VINP_EOPFVTREnableOffSta_flg/1  "VINP_EOPFVTREnableOffSta_flg"
  EOPFVTREnableOffSta/2 -> Terminator_4/1
  [BHAL_outputs] -> slr_VHAL_EOPFVTRHallSigErrSta_flg/1
  slr_VHAL_EOPFVTRHallSigErrSta_flg/1 -> EOPFVTRHallSigErrSta/1  "<VHAL_EOPFVTRHallSigErrSta_flg>"
  True_VHAL_EOPFVTRHallSigErrSta_flg/1 -> EOPFVTRHallSigErrSta/2
  [inp_CanValid_bus] -> slr1_5/1
  slr1_5/1 -> EOPFVTRHallSigErrSta/3  "<VINP_CANMsgValidEOPFVTRLocal1_flg>"
  EOPFVTRHallSigErrSta/1 -> VINP_EOPFVTRHallSigErrSta_flg/1  "VINP_EOPFVTRHallSigErrSta_flg"
  EOPFVTRHallSigErrSta/2 -> Terminator_5/1
  [BHAL_outputs] -> slr_VHAL_EOPFVTRLocal1CSSta_enum/1
  slr_VHAL_EOPFVTRLocal1CSSta_enum/1 -> EOPFVTRLocal1CSSta/1  "<VHAL_EOPFVTRLocal1CSSta_enum>"
  True_VHAL_EOPFVTRLocal1CSSta_enum/1 -> EOPFVTRLocal1CSSta/2
  [inp_CanValid_bus] -> slr1_6/1
  slr1_6/1 -> EOPFVTRLocal1CSSta/3  "<VINP_CANMsgValidEOPFVTRLocal1_flg>"
  EOPFVTRLocal1CSSta/1 -> VINP_EOPFVTRLocal1CSSta_enum/1  "VINP_EOPFVTRLocal1CSSta_enum"
  EOPFVTRLocal1CSSta/2 -> Terminator_6/1
  [BHAL_outputs] -> slr_VHAL_EOPFVTRLocal1RCSta_enum/1
  slr_VHAL_EOPFVTRLocal1RCSta_enum/1 -> EOPFVTRLocal1RCSta/1  "<VHAL_EOPFVTRLocal1RCSta_enum>"
  True_VHAL_EOPFVTRLocal1RCSta_enum/1 -> EOPFVTRLocal1RCSta/2
  [inp_CanValid_bus] -> slr1_7/1
  slr1_7/1 -> EOPFVTRLocal1RCSta/3  "<VINP_CANMsgValidEOPFVTRLocal1_flg>"
  EOPFVTRLocal1RCSta/1 -> VINP_EOPFVTRLocal1RCSta_enum/1  "VINP_EOPFVTRLocal1RCSta_enum"
  EOPFVTRLocal1RCSta/2 -> Terminator_7/1
  [BHAL_outputs] -> slr_VHAL_EOPFVTROverTempBCKSta_enum/1
  slr_VHAL_EOPFVTROverTempBCKSta_enum/1 -> EOPFVTROverTempBCKSta/1  "<VHAL_EOPFVTROverTempBCKSta_enum>"
  True_VHAL_EOPFVTROverTempBCKSta_enum/1 -> EOPFVTROverTempBCKSta/2
  [inp_CanValid_bus] -> slr1_8/1
  slr1_8/1 -> EOPFVTROverTempBCKSta/3  "<VINP_CANMsgValidEOPFVTRLocal1_flg>"
  EOPFVTROverTempBCKSta/1 -> VINP_EOPFVTROverTempBCKSta_enum/1  "VINP_EOPFVTROverTempBCKSta_enum"
  EOPFVTROverTempBCKSta/2 -> Terminator_8/1
  [BHAL_outputs] -> slr_VHAL_EOPFVTROverTempSta_flg/1
  slr_VHAL_EOPFVTROverTempSta_flg/1 -> EOPFVTROverTempSta/1  "<VHAL_EOPFVTROverTempSta_flg>"
  True_VHAL_EOPFVTROverTempSta_flg/1 -> EOPFVTROverTempSta/2
  [inp_CanValid_bus] -> slr1_9/1
  slr1_9/1 -> EOPFVTROverTempSta/3  "<VINP_CANMsgValidEOPFVTRLocal1_flg>"
  EOPFVTROverTempSta/1 -> VINP_EOPFVTROverTempSta_flg/1  "VINP_EOPFVTROverTempSta_flg"
  EOPFVTROverTempSta/2 -> Terminator_9/1
  [BHAL_outputs] -> slr_VHAL_EOPFVTROverVolSta_enum/1
  slr_VHAL_EOPFVTROverVolSta_enum/1 -> EOPFVTROverVolSta/1  "<VHAL_EOPFVTROverVolSta_enum>"
  True_VHAL_EOPFVTROverVolSta_enum/1 -> EOPFVTROverVolSta/2
  [inp_CanValid_bus] -> slr1_10/1
  slr1_10/1 -> EOPFVTROverVolSta/3  "<VINP_CANMsgValidEOPFVTRLocal1_flg>"
  EOPFVTROverVolSta/1 -> VINP_EOPFVTROverVolSta_enum/1  "VINP_EOPFVTROverVolSta_enum"
  EOPFVTROverVolSta/2 -> Terminator_10/1
  [BHAL_outputs] -> slr_VHAL_EOPFVTRPumpReadySta_flg/1
  slr_VHAL_EOPFVTRPumpReadySta_flg/1 -> EOPFVTRPumpReadySta/1  "<VHAL_EOPFVTRPumpReadySta_flg>"
  True_VHAL_EOPFVTRPumpReadySta_flg/1 -> EOPFVTRPumpReadySta/2
  [inp_CanValid_bus] -> slr1_11/1
  slr1_11/1 -> EOPFVTRPumpReadySta/3  "<VINP_CANMsgValidEOPFVTRLocal1_flg>"
  EOPFVTRPumpReadySta/1 -> VINP_EOPFVTRPumpReadySta_flg/1  "VINP_EOPFVTRPumpReadySta_flg"
  EOPFVTRPumpReadySta/2 -> Terminator_11/1
  [BHAL_outputs] -> slr_VHAL_EOPFVTRRCInvalidSta_flg/1
  slr_VHAL_EOPFVTRRCInvalidSta_flg/1 -> EOPFVTRRCInvalidSta/1  "<VHAL_EOPFVTRRCInvalidSta_flg>"
  True_VHAL_EOPFVTRRCInvalidSta_flg/1 -> EOPFVTRRCInvalidSta/2
  [inp_CanValid_bus] -> slr1_12/1
  slr1_12/1 -> EOPFVTRRCInvalidSta/3  "<VINP_CANMsgValidEOPFVTRLocal1_flg>"
  EOPFVTRRCInvalidSta/1 -> VINP_EOPFVTRRCInvalidSta_flg/1  "VINP_EOPFVTRRCInvalidSta_flg"
  EOPFVTRRCInvalidSta/2 -> Terminator_12/1
  [BHAL_outputs] -> slr_VHAL_EOPFVTRRunStatusSta_enum/1
  slr_VHAL_EOPFVTRRunStatusSta_enum/1 -> EOPFVTRRunStatusSta/1  "<VHAL_EOPFVTRRunStatusSta_enum>"
  True_VHAL_EOPFVTRRunStatusSta_enum/1 -> EOPFVTRRunStatusSta/2
  [inp_CanValid_bus] -> slr1_13/1
  slr1_13/1 -> EOPFVTRRunStatusSta/3  "<VINP_CANMsgValidEOPFVTRLocal1_flg>"
  EOPFVTRRunStatusSta/1 -> VINP_EOPFVTRRunStatusSta_enum/1  "VINP_EOPFVTRRunStatusSta_enum"
  EOPFVTRRunStatusSta/2 -> Terminator_13/1
  [BHAL_outputs] -> slr_VHAL_EOPFVTRStartFailureSta_flg/1
  slr_VHAL_EOPFVTRStartFailureSta_flg/1 -> EOPFVTRStartFailureSta/1  "<VHAL_EOPFVTRStartFailureSta_flg>"
  True_VHAL_EOPFVTRStartFailureSta_flg/1 -> EOPFVTRStartFailureSta/2
  [inp_CanValid_bus] -> slr1_14/1
  slr1_14/1 -> EOPFVTRStartFailureSta/3  "<VINP_CANMsgValidEOPFVTRLocal1_flg>"
  EOPFVTRStartFailureSta/1 -> VINP_EOPFVTRStartFailureSta_flg/1  "VINP_EOPFVTRStartFailureSta_flg"
  EOPFVTRStartFailureSta/2 -> Terminator_14/1
  [BHAL_outputs] -> slr_VHAL_EOPFVTRUnderVolSta_enum/1
  slr_VHAL_EOPFVTRUnderVolSta_enum/1 -> EOPFVTRUnderVolSta/1  "<VHAL_EOPFVTRUnderVolSta_enum>"
  True_VHAL_EOPFVTRUnderVolSta_enum/1 -> EOPFVTRUnderVolSta/2
  [inp_CanValid_bus] -> slr1_15/1
  slr1_15/1 -> EOPFVTRUnderVolSta/3  "<VINP_CANMsgValidEOPFVTRLocal1_flg>"
  EOPFVTRUnderVolSta/1 -> VINP_EOPFVTRUnderVolSta_enum/1  "VINP_EOPFVTRUnderVolSta_enum"
  EOPFVTRUnderVolSta/2 -> Terminator_15/1
